simulink model "Pitch_Simulation"  (R2022b)
settings: Solver=VariableStepAuto  StartTime=0.0  StopTime=10  RelTol=1e-3
values from neighbouring files (symbols this model uses):
  N_PitchRate_val = 20    [Pitch_Nyquist_Analysis.m]    (also in Pitch_TF_Analysis.m)
  Ts_val = 0.01    [Pitch_Nyquist_Analysis.m]    (also in Pitch_Root_Locus_Analysis.m; Pitch_TF_Analysis.m)
libraries: simulink x2
settings Model: Creator=marcv  LastModifiedBy=marcv

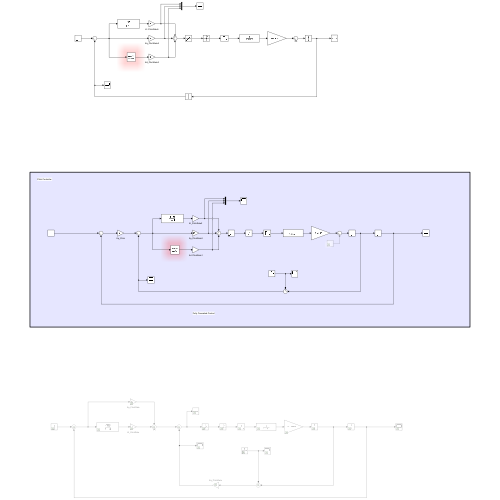
[thumbnail: Simulink's stored preview of the top-level diagram]
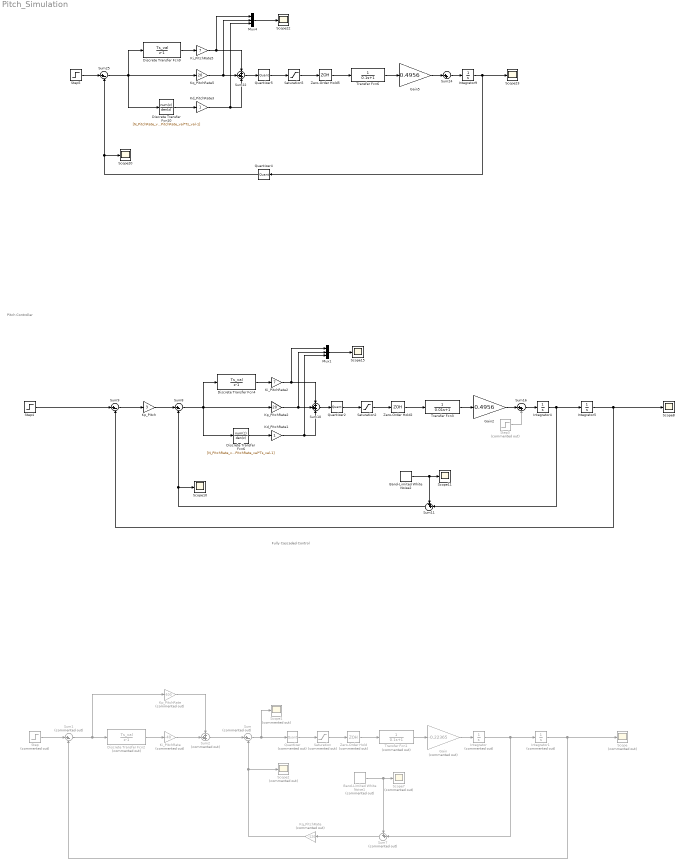
== system Pitch_Simulation ==
  note: Pitch Controller
  note: Fully Cascaded Control
  Band-Limited White Noise1 : simulink/Sources/Band-Limited White Noise  Commented=on  Cov=1e-9  Ts=Ts_val  seed=[23341]
  Band-Limited White Noise2 : simulink/Sources/Band-Limited White Noise  Cov=1e-6  Ts=Ts_val  seed=[23341]
  Discrete Transfer Fcn10 : DiscreteTransferFcn  Numerator=[N_PitchRate_val, -N_PitchRate_val]  Denominator=[1, N_PitchRate_val*Ts_val-1]  SampleTime=Ts_val
  Discrete Transfer Fcn2 : DiscreteTransferFcn  Commented=on  Numerator=Ts_val  Denominator=[1,-1]  SampleTime=Ts_val
  Discrete Transfer Fcn4 : DiscreteTransferFcn  Numerator=Ts_val  Denominator=[1,-1]  SampleTime=Ts_val
  Discrete Transfer Fcn6 : DiscreteTransferFcn  Numerator=[N_PitchRate_val, -N_PitchRate_val]  Denominator=[1, N_PitchRate_val*Ts_val-1]  SampleTime=Ts_val
  Discrete Transfer Fcn9 : DiscreteTransferFcn  Numerator=Ts_val  Denominator=[1,-1]  SampleTime=Ts_val
  Gain : Gain  Commented=on  Gain=-0.22365
  Gain2 : Gain  Gain=0.4956
  Gain5 : Gain  Gain=0.4956
  Integrator : Integrator  Commented=on
  Integrator1 : Integrator  Commented=on
  Integrator4 : Integrator
  Integrator5 : Integrator
  Integrator9 : Integrator
  Kd_PitchRate1 : Gain
  Kd_PitchRate3 : Gain
  Ki_PitchRate : Gain  Commented=on  Gain=-40
  Ki_PitchRate2 : Gain  Gain=7
  Ki_PitchRate5 : Gain  Gain=7
  Kp_Pitch : Gain  Gain=3
  Kp_PitchRate : Gain  Commented=on  Gain=-500
  Kp_PitchRate2 : Gain  Gain=20
  Kq_PitchRate : Gain  Commented=on  Gain=-120
  Kq_PitchRate5 : Gain  Gain=20
  Mux1 : Mux  Inputs=3
  Mux4 : Mux  Inputs=3
  Quantizer : Quantizer  Commented=on  QuantizationInterval=5
  Quantizer2 : Quantizer  QuantizationInterval=1
  Quantizer4 : Quantizer  QuantizationInterval=0.001
  Quantizer5 : Quantizer  QuantizationInterval=1
  Saturation : Saturate  Commented=on  UpperLimit=200  LowerLimit=-200
  Saturation2 : Saturate  UpperLimit=200  LowerLimit=-200
  Saturation5 : Saturate  UpperLimit=200  LowerLimit=-200
  Scope{,1..2,7} (4 alike) : Scope  Commented=on
  Scope{8,10..11,15,20,22..23} (7 alike) : Scope
  Step : Step  Commented=on  SampleTime=0
  Step3 : Step  Commented=on  SampleTime=0
  Step4 : Step  After=0.25  SampleTime=0
  Step5 : Step  SampleTime=0
  Sum : Sum  Commented=on  Inputs=|+-
  Sum1 : Sum  Commented=on  Inputs=|+-
  Sum10 : Sum  Inputs=+++
  Sum11 : Sum  Inputs=++|
  Sum16 : Sum  Inputs=|++
  Sum2 : Sum  Commented=on  Inputs=+++
  Sum22 : Sum  Inputs=+++
  Sum24 : Sum  Inputs=|++
  Sum25 : Sum  Inputs=|+-
  Sum7 : Sum  Commented=on  Inputs=++|
  Sum8 : Sum  Inputs=|+-
  Sum9 : Sum  Inputs=|+-
  Transfer Fcn1 : TransferFcn  Commented=on  Denominator=[0.1 1]
  Transfer Fcn3 : TransferFcn  Denominator=[0.01 1]
  Transfer Fcn6 : TransferFcn  Denominator=[0.1 1]
  Zero-Order Hold : ZeroOrderHold  Commented=on  SampleTime=Ts_val
  Zero-Order Hold2 : ZeroOrderHold  SampleTime=Ts_val
  Zero-Order Hold5 : ZeroOrderHold  SampleTime=Ts_val
  wires:
  Zero-Order Hold/1 -> Transfer Fcn1/1
  Gain/1 -> Integrator/1
  Integrator/1 -> Sum7/2, Integrator1/1
  Integrator1/1 -> Scope/1, Sum1/2
  Step/1 -> Sum1/1
  Ki_PitchRate/1 -> Sum2/2
  Kp_PitchRate/1 -> Sum2/1
  Discrete Transfer Fcn2/1 -> Ki_PitchRate/1
  Quantizer/1 -> Saturation/1
  Saturation/1 -> Zero-Order Hold/1
  Sum/1 -> Scope1/1, Quantizer/1
  Sum2/1 -> Sum/1
  Kq_PitchRate/1 -> Scope2/1, Sum/2
  Transfer Fcn1/1 -> Gain/1
  Sum1/1 -> Kp_PitchRate/1, Discrete Transfer Fcn2/1
  Band-Limited White Noise1/1 -> Scope7/1, Sum7/1
  Sum7/1 -> Kq_PitchRate/1
  Band-Limited White Noise2/1 -> Scope11/1, Sum11/1
  Transfer Fcn3/1 -> Gain2/1
  Step4/1 -> Sum9/1
  Integrator4/1 -> Sum11/2, Integrator5/1
  Integrator5/1 -> Scope8/1, Sum9/2
  Kp_Pitch/1 -> Sum8/1
  Discrete Transfer Fcn4/1 -> Ki_PitchRate2/1
  Sum9/1 -> Kp_Pitch/1
  Sum8/1 -> Discrete Transfer Fcn6/1, Kp_PitchRate2/1, Discrete Transfer Fcn4/1
  Discrete Transfer Fcn6/1 -> Kd_PitchRate1/1
  Gain2/1 -> Sum16/1
  Sum16/1 -> Integrator4/1
  Kd_PitchRate1/1 -> Mux1/3, Sum10/3
  Kp_PitchRate2/1 -> Mux1/2, Sum10/2
  Mux1/1 -> Scope15/1
  Ki_PitchRate2/1 -> Sum10/1, Mux1/1
  Sum25/1 -> Discrete Transfer Fcn10/1, Kq_PitchRate5/1, Discrete Transfer Fcn9/1
  Integrator9/1 -> Quantizer4/1, Scope23/1
  Kq_PitchRate5/1 -> Mux4/2, Sum22/2
  Kd_PitchRate3/1 -> Mux4/3, Sum22/3
  Discrete Transfer Fcn9/1 -> Ki_PitchRate5/1
  Gain5/1 -> Sum24/1
  Mux4/1 -> Scope22/1
  Ki_PitchRate5/1 -> Sum22/1, Mux4/1
  Discrete Transfer Fcn10/1 -> Kd_PitchRate3/1
  Sum24/1 -> Integrator9/1
  Step5/1 -> Sum25/1
  Transfer Fcn6/1 -> Gain5/1
  Zero-Order Hold5/1 -> Transfer Fcn6/1
  Saturation5/1 -> Zero-Order Hold5/1
  Sum22/1 -> Quantizer5/1
  Step3/1 -> Sum16/2
  Quantizer2/1 -> Saturation2/1
  Saturation2/1 -> Zero-Order Hold2/1
  Sum11/1 -> Sum8/2, Scope10/1
  Quantizer5/1 -> Saturation5/1
  Quantizer4/1 -> Sum25/2, Scope20/1
  Sum10/1 -> Quantizer2/1
  Zero-Order Hold2/1 -> Transfer Fcn3/1
